simulink library "nav_lib"  (R2023b)
settings: Solver=VariableStepAuto  StartTime=0.0  StopTime=10.0  RelTol=1e-3
values from neighbouring files (symbols this model uses):
  Q = Q + (obj.ref_radius/obj.r)^n*Qn    [SH_gradient.m]    (also in SH_nav.m = Q + reorn * Q_n)
undefined symbols (not defined in the file or in its folder): BeaconSpacecraft, Environment, MainSpacecraft, mu_m, Propagation, R_sensor2body, StartDate, x0
libraries: dyn_lib x14, matrix_library x9, $bdroot x7, simulink x4, vrlib x2
(part 2 of 2)

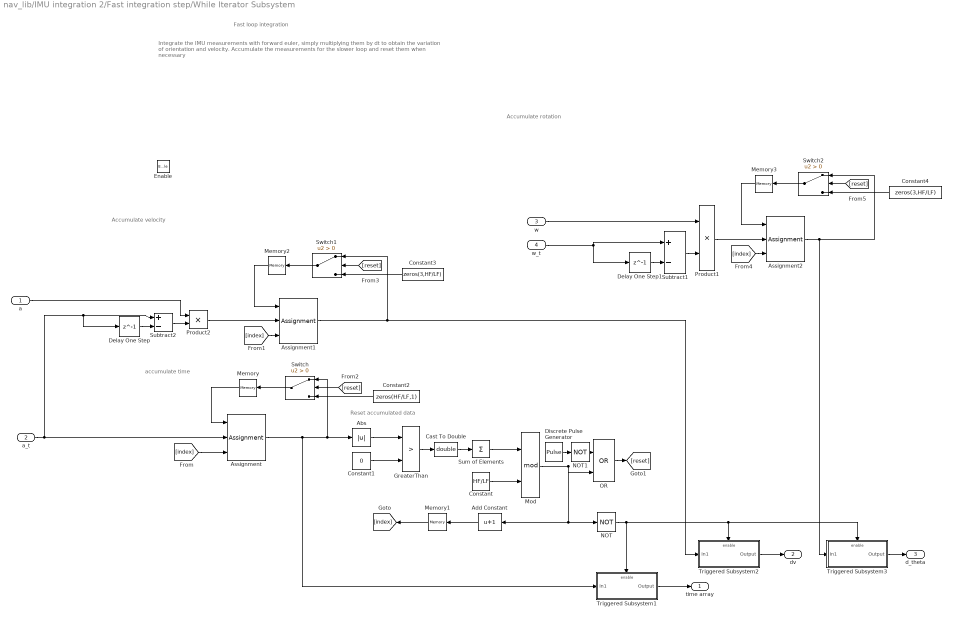
== system nav_lib/IMU integration 2/Fast integration step/While Iterator Subsystem ==
  note: Integrate the IMU measurements with forward euler, simply multiplying them by dt to obtain the variation of orientation and velocity. Accumulate the measurements for the slower loop and reset them when necessary
  note: Fast loop integration
  note: Reset accumulated data
  note: accumulate time
  note: Accumulate velocity
  note: Accumulate rotation
  a : Inport
  a_t : Inport  Port=2
  w : Inport  Port=3
  w_t : Inport  Port=4
  Enable : EnablePort  PropagateVarSize=During execution
  Abs : Abs  SaturateOnIntegerOverflow=off
  Add Constant : Bias  Bias=1  SaturateOnIntegerOverflow=off
  Assignment : Assignment  NumberOfDimensions=2  DiagnosticForDimensions=Warning  IndexOptions=Index vector (port),Index vector (dialog)  Indices=1,1  OutputSizes=1,1
  Assignment1 : Assignment  NumberOfDimensions=2  DiagnosticForDimensions=Warning  IndexOptions=Assign all,Index vector (port)  Indices=1,1  OutputSizes=1,1
  Assignment2 : Assignment  NumberOfDimensions=2  DiagnosticForDimensions=Warning  IndexOptions=Assign all,Index vector (port)  Indices=1,1  OutputSizes=1,1
  Cast To Double : DataTypeConversion  OutDataTypeStr=double  SaturateOnIntegerOverflow=off  RndMeth=Floor
  Constant : Constant  Value=HF/LF
  Constant1 : Constant  Value=0
  Constant2 : Constant  Value=zeros(HF/LF,1)  VectorParams1D=off
  Constant3 : Constant  Value=zeros(3,HF/LF)  VectorParams1D=off
  Constant4 : Constant  Value=zeros(3,HF/LF)  VectorParams1D=off
  Delay One Step : Delay  DelayLength=1  InitialCondition=0
  Delay One Step1 : Delay  DelayLength=1  InitialCondition=0
  Discrete Pulse Generator : DiscretePulseGenerator  Period=HF/LF  SampleTime=1/HF
  GreaterThan : RelationalOperator  Operator=>  OutDataTypeStr=boolean  RndMeth=Simplest  InputSameDT=off
  Memory : Memory  InitialCondition=zeros(HF/LF,1)  InheritSampleTime=on
  Memory1 : Memory  InitialCondition=1  InheritSampleTime=on
  Memory2 : Memory  InitialCondition=zeros(3,6)  InheritSampleTime=on
  Memory3 : Memory  InitialCondition=zeros(3,HF/LF)  InheritSampleTime=on
  Mod : Math  Operator=mod
  NOT : Logic  Operator=NOT  IconShape=distinctive  AllPortsSameDT=off  OutDataTypeStr=boolean
  NOT1 : Logic  Operator=NOT  IconShape=distinctive  AllPortsSameDT=off  OutDataTypeStr=boolean
  OR : Logic  Operator=OR  IconShape=distinctive  AllPortsSameDT=off  OutDataTypeStr=boolean
  Product1 : Product
  Product2 : Product
  Subtract1 : Sum  Inputs=+-
  Subtract2 : Sum  Inputs=+-
  Sum of Elements : Sum  Inputs=+
  Switch : Switch  Criteria=u2 > Threshold  SaturateOnIntegerOverflow=off  InputSameDT=off
  Switch1 : Switch  Criteria=u2 > Threshold  SaturateOnIntegerOverflow=off  InputSameDT=off
  Switch2 : Switch  Criteria=u2 > Threshold  SaturateOnIntegerOverflow=off  InputSameDT=off
  Triggered Subsystem1 : Subsystem  TreatAsAtomicUnit=on
  Triggered Subsystem2 : Subsystem  TreatAsAtomicUnit=on
  Triggered Subsystem3 : Subsystem  TreatAsAtomicUnit=on
  time array : Outport
  dv : Outport  Port=2
  d_theta : Outport  Port=3
  wires:
  NOT1/1 -> OR/1
  Discrete Pulse Generator/1 -> NOT1/1
  OR/1 -> [reset]
  Subtract2/1 -> Product2/2
  a_t/1 -> Subtract2/1, Delay One Step/1, Assignment/2
  a/1 -> Product2/1
  Delay One Step/1 -> Subtract2/2
  Memory/1 -> Assignment/1
  Constant1/1 -> GreaterThan/2
  Abs/1 -> GreaterThan/1
  GreaterThan/1 -> Cast To Double/1
  Constant/1 -> Mod/2
  Sum of Elements/1 -> Mod/1
  Cast To Double/1 -> Sum of Elements/1
  Add Constant/1 -> Memory1/1
  Switch/1 -> Memory/1
  Mod/1 -> OR/2, NOT/1, Add Constant/1
  Constant2/1 -> Switch/3
  Assignment/1 -> Triggered Subsystem1/1(In1), Switch/1, Abs/1
  Triggered Subsystem1/1(Output) -> time array/1
  NOT/1 -> Triggered Subsystem3/Enable, Triggered Subsystem2/Enable, Triggered Subsystem1/Enable
  Memory1/1 -> [index]
  [index] -> Assignment/3
  Switch1/1 -> Memory2/1
  Memory2/1 -> Assignment1/1
  Product2/1 -> Assignment1/2
  [index] -> Assignment1/3
  Assignment1/1 -> Triggered Subsystem2/1(In1), Switch1/1
  Constant3/1 -> Switch1/3
  Triggered Subsystem2/1(Output) -> dv/1
  [reset] -> Switch/2
  [reset] -> Switch1/2
  Subtract1/1 -> Product1/2
  Delay One Step1/1 -> Subtract1/2
  w_t/1 -> Delay One Step1/1, Subtract1/1
  w/1 -> Product1/1
  Constant4/1 -> Switch2/3
  Switch2/1 -> Memory3/1
  [reset] -> Switch2/2
  Product1/1 -> Assignment2/2
  Memory3/1 -> Assignment2/1
  [index] -> Assignment2/3
  Assignment2/1 -> Triggered Subsystem3/1(In1), Switch2/1
  Triggered Subsystem3/1(Output) -> d_theta/1

== system nav_lib/IMU integration 2/gyro integration/No rotation ==
  q_k-1 : Inport
  Enable : EnablePort
  q_k : Outport
  wires:
  q_k-1/1 -> q_k/1

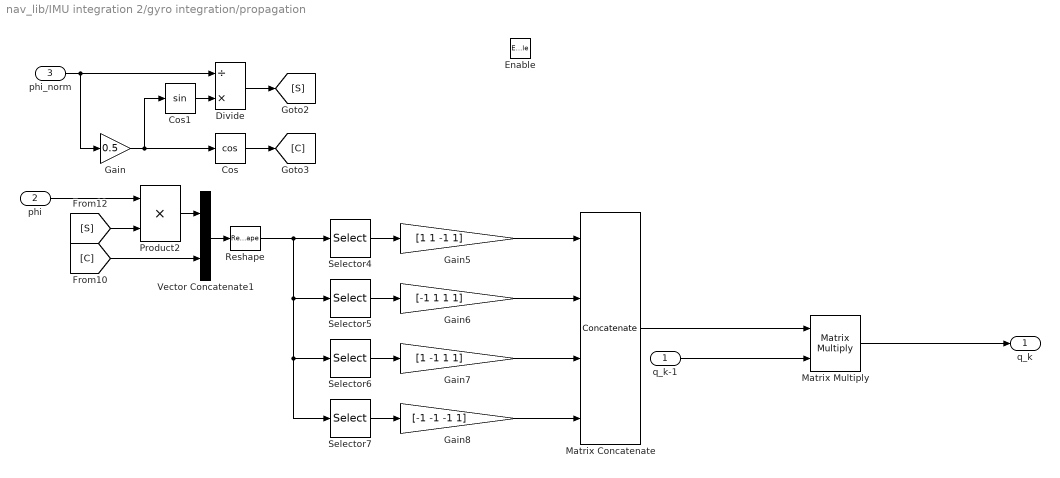
== system nav_lib/IMU integration 2/gyro integration/propagation ==
  q_k-1 : Inport
  phi : Inport  Port=2
  phi_norm : Inport  Port=3
  Enable : EnablePort
  Cos : Trigonometry  Operator=cos  OutputSignalType=real
  Cos1 : Trigonometry  OutputSignalType=real
  Divide : Product  Inputs=/*
  Gain : Gain  Gain=0.5
  Gain5 : Gain  Gain=[1 1 -1 1]
  Gain6 : Gain  Gain=[-1 1 1 1]
  Gain7 : Gain  Gain=[1 -1 1 1]
  Gain8 : Gain  Gain=[-1 -1 -1 1]
  Matrix Concatenate : Concatenate  NumInputs=4  Mode=Multidimensional array
  Matrix Multiply : Product  Multiplication=Matrix(*)
  Product2 : Product
  Reshape : Reshape  OutputDimensionality=Row vector (2-D)
  Selector4 : Selector  InputPortWidth=4  IndexOptions=Index vector (dialog)  Indices=[4 3 2 1]  OutputSizes=1
  Selector5 : Selector  InputPortWidth=4  IndexOptions=Index vector (dialog)  Indices=[3 4 1 2]  OutputSizes=1
  Selector6 : Selector  InputPortWidth=4  IndexOptions=Index vector (dialog)  Indices=[2 1 4 3]  OutputSizes=1
  Selector7 : Selector  InputPortWidth=4  IndexOptions=Index vector (dialog)  Indices=[1 2 3 4]  OutputSizes=1
  Vector Concatenate1 : Concatenate
  q_k : Outport
  wires:
  [C] -> Vector Concatenate1/2
  Gain5/1 -> Matrix Concatenate/1
  Gain/1 -> Cos1/1, Cos/1
  Gain7/1 -> Matrix Concatenate/3
  Selector5/1 -> Gain6/1
  Matrix Multiply/1 -> q_k/1
  Cos1/1 -> Divide/2
  Divide/1 -> [S]
  phi/1 -> Product2/1
  Gain6/1 -> Matrix Concatenate/2
  Vector Concatenate1/1 -> Reshape/1
  [S] -> Product2/2
  Selector6/1 -> Gain7/1
  Selector7/1 -> Gain8/1
  Selector4/1 -> Gain5/1
  phi_norm/1 -> Divide/1, Gain/1
  Cos/1 -> [C]
  Matrix Concatenate/1 -> Matrix Multiply/1
  Reshape/1 -> Selector7/1, Selector6/1, Selector5/1, Selector4/1
  q_k-1/1 -> Matrix Multiply/2
  Product2/1 -> Vector Concatenate1/1
  Gain8/1 -> Matrix Concatenate/4

== system nav_lib/IMU integration 2/Fast integration step/While Iterator Subsystem/Triggered Subsystem1 ==
  In1 : Inport
  Enable : EnablePort
  Output : Outport
  wires:
  In1/1 -> Output/1

== system nav_lib/IMU integration 2/Fast integration step/While Iterator Subsystem/Triggered Subsystem2 ==
  In1 : Inport
  Enable : EnablePort
  Output : Outport
  wires:
  In1/1 -> Output/1

== system nav_lib/IMU integration 2/Fast integration step/While Iterator Subsystem/Triggered Subsystem3 ==
  In1 : Inport
  Enable : EnablePort
  Output : Outport
  wires:
  In1/1 -> Output/1
